simulink model "r2sdf_fft_blk"  (R2018a)
settings: Solver=VariableStepAuto  StartTime=0.0  StopTime=10.0  RelTol=1e-3
libraries: xbsIndex_r4 x1
settings Model: Creator=talon  LastModifiedBy=talonm
settings DataIOCC: ReturnWorkspaceOutputs=on
settings SFSimCC: SimUseLocalCustomCode=on
settings RTWCC: RTWUseLocalCustomCode=on

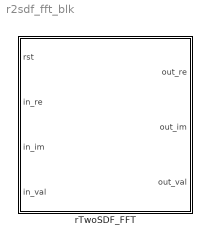
== system r2sdf_fft_blk ==
  rTwoSDF_FFT : Subsystem  mask{g_nof_chan=0, g_use_reorder=on, g_in_dat_w=8, g_out_dat_w=14, g_stage_dat_w=18, g_guard_w=2, g_nof_points=512, g_variant="4DSP", g_use_dsp="yes", g_technology=0, g_ram_primitive="auto"}
      mask prompts: g_nof_chan "Number of channels"; g_use_reorder "Reorder output"; g_in_dat_w "Input data width"; g_out_dat_w "Output data width"; g_stage_dat_w "Stage data width"; g_guard_w "Guard bit width"; g_nof_points "Number of points"; g_variant "3 or 4 DSP for cmults"; g_use_dsp "Use DSP for cmults"; g_technology "Vendor (0-Xilinx, 1-Alterra)"; g_ram_primitive "Ram Primitive"
      mask TypeOptions g_variant: "3DSP" | "4DSP"
      mask TypeOptions g_use_dsp: "yes" | "no"
      mask TypeOptions g_technology: 0 | 1
      mask TypeOptions g_ram_primitive: "auto" | "distributed" | "block" | "ultra"

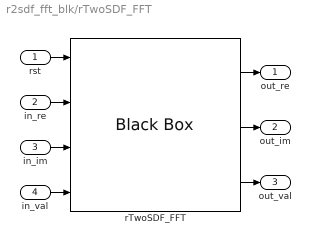
== system r2sdf_fft_blk/rTwoSDF_FFT ==
  rst : Inport
  in_re : Inport  Port=2
  in_im : Inport  Port=3
  in_val : Inport  Port=4
  rTwoSDF_FFT : xbsIndex_r4/Black Box  init_code=rTwoSDF_config  sim_method=ISE Simulator  verbose=off  block_type=blackbox2
  out_re : Outport
  out_im : Outport  Port=2
  out_val : Outport  Port=3
  wires:
  rTwoSDF_FFT/3 -> out_val/1
  in_im/1 -> rTwoSDF_FFT/3
  rst/1 -> rTwoSDF_FFT/1
  rTwoSDF_FFT/2 -> out_im/1
  in_re/1 -> rTwoSDF_FFT/2
  in_val/1 -> rTwoSDF_FFT/4
  rTwoSDF_FFT/1 -> out_re/1
